simulink model "SerialCommIn_V2"  (R2017b)
settings: Solver=FixedStepAuto  StartTime=0.0  StopTime=inf  FixedStep=0.001  RelTol=1e-3  EnableMultiTasking=on
undefined symbols (not defined in the file): D10, D11, D12, D2, D5, D8, D9, PTA0, PTA2, PTB9, PTC4, PTD0, PTD2, PTD3
libraries: frdmk64flib x22, etargetslib x1
settings Model: ExtModeTrigDuration=5  Creator=montema2  LastModifiedBy=farona
settings OptimizationCC: PassReuseOutputArgsAs=Individual arguments  MaxStackSize=64
settings DebuggingCC: ParameterTunabilityLossMsg=error
settings HardwareCC: ProdBitPerPointer=32  ProdBitPerSizeT=32  ProdBitPerPtrDiffT=32  ProdLargestAtomicInteger=Long  ProdLargestAtomicFloat=Double  ProdWordSize=32  ProdHWDeviceType=ARM Compatible->ARM Cortex
settings SFSimCC: MATLABDynamicMemAlloc=off
settings RTWCC: SystemTargetFile=ert.tlc  HardwareBoard=NXP FRDM-K64F  TemplateMakefile=ert_default_tmf  GenerateReport=on  Toolchain=GNU Tools for ARM Embedded Processors  IncludeHyperlinkInReport=on  LaunchReport=on  GenerateTraceInfo=on  GenerateTraceReport=on  GenerateTraceReportSl=on  GenerateTraceReportSf=on  GenerateTraceReportEml=on
settings CodeAppCC: ForceParamTrailComments=on  IgnoreCustomStorageClasses=off  OperatorAnnotations=on  SimulinkDataObjDesc=on  SFDataObjDesc=on  InsertBlockDesc=on

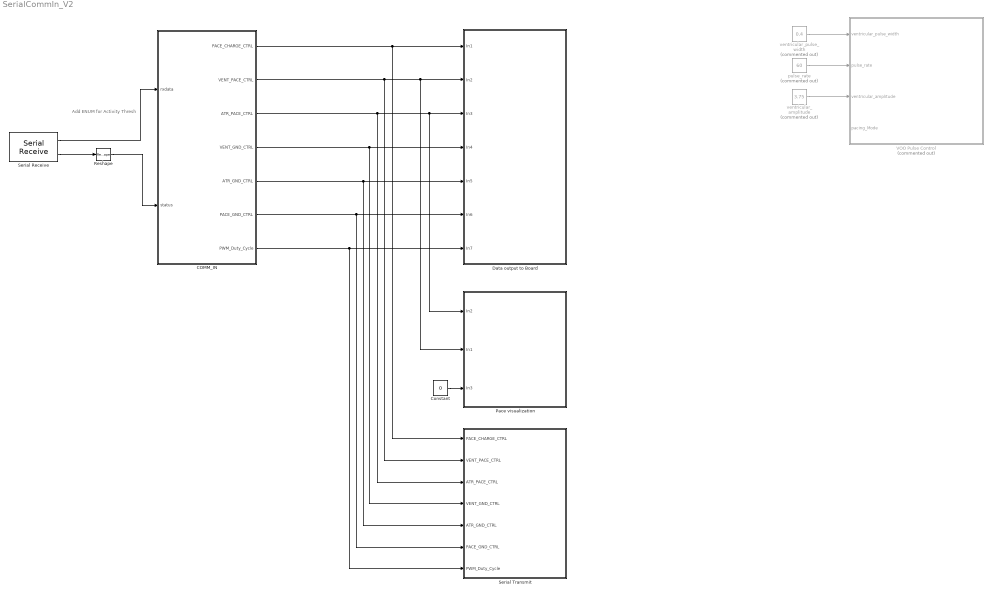
== system SerialCommIn_V2 ==
  note: Add ENUM for Activity Thresh
  COMM_IN : Stateflow chart  TreatAsAtomicUnit=on
  Constant : Constant  Value=0
  Data output to Board : Subsystem
  Pace visualization : Subsystem
  Reshape : Reshape  OutputDimensionality=Customize  OutputDimensions=[1]
  Serial Receive : frdmk64flib/Serial Receive  SCIModule=0  Baudrate=uint32(9600)  Parity=None  StopBits=1  HardwareFlowControl=None  ByteOrder=LittleEndian  DataType=uint8  DataLength=31  BlockingMode=off  OutputStatus=on  SampleTime=-1
      settings: SourceProductName=Simulink Coder Support Package for NXP FRDM-K64F Board
  Serial Transmit : Subsystem
  VOO Pulse Control : Subsystem  Commented=on
  pulse_rate : Constant  Commented=on  Value=60  OutMin=[50]  OutMax=[175]
  ventricular_amplitude : Constant  Commented=on  Value=3.75
  ventricular_pulse_width : Constant  Commented=on  Value=0.4
  wires:
  ventricular_pulse_width/1 -> VOO Pulse Control/1(ventricular_pulse_width)
  pulse_rate/1 -> VOO Pulse Control/2(pulse_rate)
  ventricular_amplitude/1 -> VOO Pulse Control/3(ventricular_amplitude)
  Serial Receive/2 -> Reshape/1
  COMM_IN/4(VENT_GND_CTRL) -> Serial Transmit/4(VENT_GND_CTRL), Data output to Board/4(In4)
  COMM_IN/6(PACE_GND_CTRL) -> Serial Transmit/6(PACE_GND_CTRL), Data output to Board/6(In6)
  COMM_IN/1(PACE_CHARGE_CTRL) -> Serial Transmit/1(PACE_CHARGE_CTRL), Data output to Board/1(In1)
  COMM_IN/7(PWM_Duty_Cycle) -> Serial Transmit/7(PWM_Duty_Cycle), Data output to Board/7(In7)
  COMM_IN/5(ATR_GND_CTRL) -> Serial Transmit/5(ATR_GND_CTRL), Data output to Board/5(In5)
  COMM_IN/2(VENT_PACE_CTRL) -> Serial Transmit/2(VENT_PACE_CTRL), Pace visualization/2(In1), Data output to Board/2(In2)
  COMM_IN/3(ATR_PACE_CTRL) -> Serial Transmit/3(ATR_PACE_CTRL), Pace visualization/1(In2), Data output to Board/3(In3)
  Serial Receive/1 -> COMM_IN/1(rxdata)
  Constant/1 -> Pace visualization/3(In3)
  Reshape/1 -> COMM_IN/2(status)

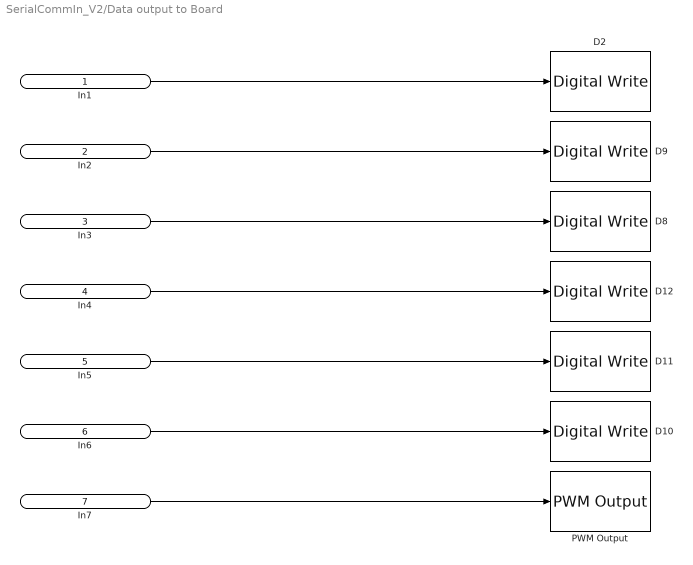
== system SerialCommIn_V2/Data output to Board ==
  In1 : Inport
  In2 : Inport  Port=2
  In3 : Inport  Port=3
  In4 : Inport  Port=4
  In5 : Inport  Port=5
  In6 : Inport  Port=6
  In7 : Inport  Port=7
  D10 : frdmk64flib/Digital Write  Whichpin=PTD0 (D10)
      settings: SourceProductName=Simulink Coder Support Package for NXP FRDM-K64F Board
  D11 : frdmk64flib/Digital Write  Whichpin=PTD2 (D11)
      settings: SourceProductName=Simulink Coder Support Package for NXP FRDM-K64F Board
  D12 : frdmk64flib/Digital Write  Whichpin=PTD3 (D12)
      settings: SourceProductName=Simulink Coder Support Package for NXP FRDM-K64F Board
  D2 : frdmk64flib/Digital Write  Whichpin=PTB9 (D2)
      settings: SourceProductName=Simulink Coder Support Package for NXP FRDM-K64F Board
  D8 : frdmk64flib/Digital Write  Whichpin=PTA0 (D8)
      settings: SourceProductName=Simulink Coder Support Package for NXP FRDM-K64F Board
  D9 : frdmk64flib/Digital Write  Whichpin=PTC4 (D9)
      settings: SourceProductName=Simulink Coder Support Package for NXP FRDM-K64F Board
  PWM Output : frdmk64flib/PWM Output  Whichpin=PTA2 (D5)  InitialFrequency=1000  InitialDutyCycle=0
      settings: SourceProductName=Simulink Coder Support Package for NXP FRDM-K64F Board
  wires:
  In1/1 -> D2/1
  In6/1 -> D10/1
  In2/1 -> D9/1
  In4/1 -> D12/1
  In3/1 -> D8/1
  In7/1 -> PWM Output/1
  In5/1 -> D11/1

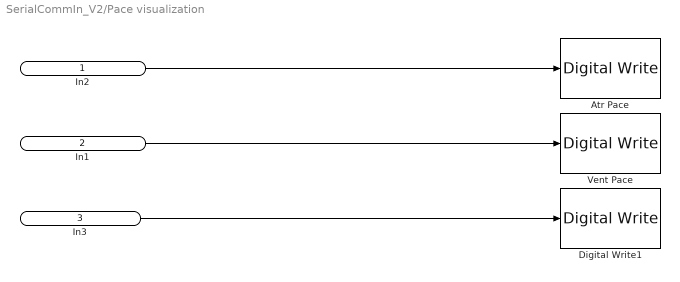
== system SerialCommIn_V2/Pace visualization ==
  In2 : Inport
  In1 : Inport  Port=2
  In3 : Inport  Port=3
  Atr Pace : frdmk64flib/Digital Write  Whichpin=GREEN_LED
      settings: SourceProductName=Simulink Coder Support Package for NXP FRDM-K64F Board
  Digital Write1 : frdmk64flib/Digital Write  Whichpin=BLUE_LED
      settings: SourceProductName=Simulink Coder Support Package for NXP FRDM-K64F Board
  Vent Pace : frdmk64flib/Digital Write  Whichpin=RED_LED
      settings: SourceProductName=Simulink Coder Support Package for NXP FRDM-K64F Board
  wires:
  In3/1 -> Digital Write1/1
  In2/1 -> Atr Pace/1
  In1/1 -> Vent Pace/1

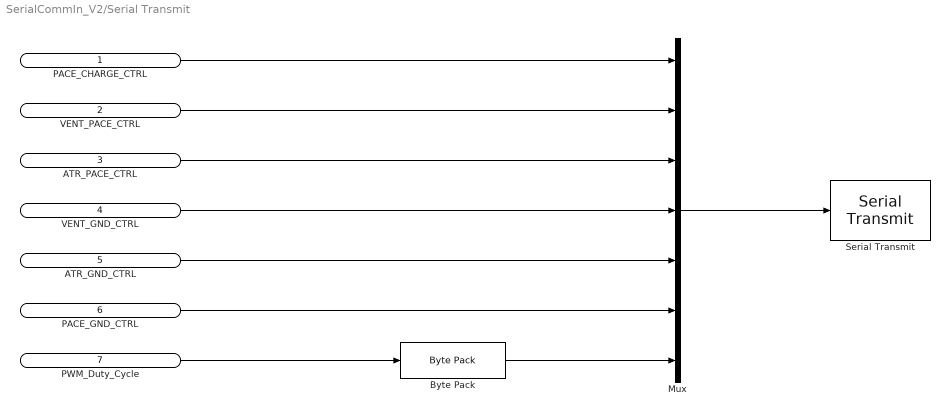
== system SerialCommIn_V2/Serial Transmit ==
  PACE_CHARGE_CTRL : Inport  OutDataTypeStr=boolean
  VENT_PACE_CTRL : Inport  Port=2  OutDataTypeStr=boolean
  ATR_PACE_CTRL : Inport  Port=3  OutDataTypeStr=boolean
  VENT_GND_CTRL : Inport  Port=4  OutDataTypeStr=boolean
  ATR_GND_CTRL : Inport  Port=5  OutDataTypeStr=boolean
  PACE_GND_CTRL : Inport  Port=6  OutDataTypeStr=boolean
  PWM_Duty_Cycle : Inport  Port=7  OutDataTypeStr=double
  Byte Pack : etargetslib/Byte Pack  datatypes={'double'}  byteAlign=1
  Mux : Mux  Inputs=7
  Serial Transmit : frdmk64flib/Serial Transmit  SCIModule=0  Baudrate=uint32(9600)  Parity=None  StopBits=1  HardwareFlowControl=None  ByteOrder=LittleEndian  BlockingMode=on  OutputStatus=off
      settings: SourceProductName=Simulink Coder Support Package for NXP FRDM-K64F Board
  wires:
  Mux/1 -> Serial Transmit/1
  PACE_CHARGE_CTRL/1 -> Mux/1
  VENT_PACE_CTRL/1 -> Mux/2
  ATR_PACE_CTRL/1 -> Mux/3
  VENT_GND_CTRL/1 -> Mux/4
  ATR_GND_CTRL/1 -> Mux/5
  PACE_GND_CTRL/1 -> Mux/6
  PWM_Duty_Cycle/1 -> Byte Pack/1
  Byte Pack/1 -> Mux/7

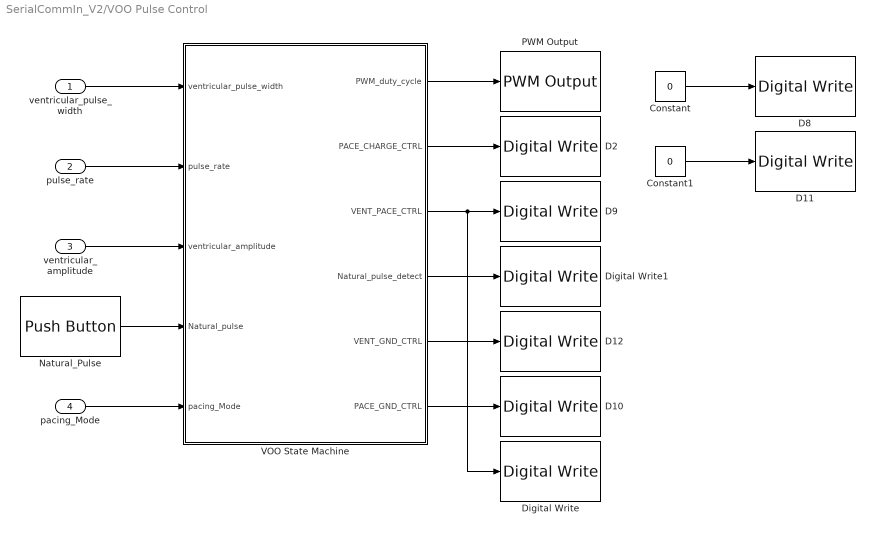
== system SerialCommIn_V2/VOO Pulse Control ==
  ventricular_pulse_width : Inport
  pulse_rate : Inport  Port=2
  ventricular_amplitude : Inport  Port=3
  pacing_Mode : Inport  Port=4
  Constant : Constant  Value=0
  Constant1 : Constant  Value=0
  D10 : frdmk64flib/Digital Write  Whichpin=PTD0 (D10)
      settings: SourceProductName=Simulink Coder Support Package for NXP FRDM-K64F Board
  D11 : frdmk64flib/Digital Write  Whichpin=PTD2 (D11)
      settings: SourceProductName=Simulink Coder Support Package for NXP FRDM-K64F Board
  D12 : frdmk64flib/Digital Write  Whichpin=PTD3 (D12)
      settings: SourceProductName=Simulink Coder Support Package for NXP FRDM-K64F Board
  D2 : frdmk64flib/Digital Write  Whichpin=PTB9 (D2)
      settings: SourceProductName=Simulink Coder Support Package for NXP FRDM-K64F Board
  D8 : frdmk64flib/Digital Write  Whichpin=PTA0 (D8)
      settings: SourceProductName=Simulink Coder Support Package for NXP FRDM-K64F Board
  D9 : frdmk64flib/Digital Write  Whichpin=PTC4 (D9)
      settings: SourceProductName=Simulink Coder Support Package for NXP FRDM-K64F Board
  Digital Write : frdmk64flib/Digital Write  Whichpin=RED_LED
      settings: SourceProductName=Simulink Coder Support Package for NXP FRDM-K64F Board
  Digital Write1 : frdmk64flib/Digital Write  Whichpin=BLUE_LED
      settings: SourceProductName=Simulink Coder Support Package for NXP FRDM-K64F Board
  Natural_Pulse : frdmk64flib/Push Button  Whichswitch=SW2  SampleTime1=-1
      settings: SourceProductName=Simulink Coder Support Package for NXP FRDM-K64F Board
  PWM Output : frdmk64flib/PWM Output  Whichpin=PTA2 (D5)  InitialFrequency=1000  InitialDutyCycle=0
      settings: SourceProductName=Simulink Coder Support Package for NXP FRDM-K64F Board
  VOO State Machine : Stateflow chart  TreatAsAtomicUnit=on
  wires:
  ventricular_pulse_width/1 -> VOO State Machine/1(ventricular_pulse_width)
  VOO State Machine/1(PWM_duty_cycle) -> PWM Output/1
  VOO State Machine/3(VENT_PACE_CTRL) -> Digital Write/1, D9/1
  pulse_rate/1 -> VOO State Machine/2(pulse_rate)
  VOO State Machine/2(PACE_CHARGE_CTRL) -> D2/1
  VOO State Machine/5(VENT_GND_CTRL) -> D12/1
  VOO State Machine/6(PACE_GND_CTRL) -> D10/1
  Constant/1 -> D8/1
  Constant1/1 -> D11/1
  Natural_Pulse/1 -> VOO State Machine/4(Natural_pulse)
  VOO State Machine/4(Natural_pulse_detect) -> Digital Write1/1
  ventricular_amplitude/1 -> VOO State Machine/3(ventricular_amplitude)
  pacing_Mode/1 -> VOO State Machine/5(pacing_Mode)

== stateflow chart SerialCommIn_V2/COMM_IN ==
  state INITIAL
    %Set intial values of parameters
    %VOO mode?
    entry: rateAdapt = 0;
    vent_Pulse_Width = 10; %milliseconds
    atr_Pulse_Width = 10;
    min_Rate_Lim = 60; %bpm
    vent_Pulse_Amp = 3.5; %volts
    atr_Pulse_Amp = 3.5;
  state VENT_CURRENT_IN
    entry:PWM_Duty_Cycle = vent_Pulse_Amp;
    PACE_CHARGE_CTRL=false;
    VENT_GND_CTRL=false;
    VENT_PACE_CTRL=true;
  state STANDBY
    %Wait for signal from DCM
  state VENTRICLE_INIT
    entry:VENT_PACE_CTRL=false;
    VENT_GND_CTRL=true;
    ATR_PACE_CTRL=false;
    ATR_GND_CTRL=true;
    PACE_CHARGE_CTRL=true;
    PACE_GND_CTRL=true;
  note: double check ATR_GND_CTRL state
  state VENT_PULSE_SENSE [commented out]
  note: double check VENT_GND_CTRL state
  state ATRIAL_INIT
    entry:VENT_PACE_CTRL=false;
    VENT_GND_CTRL=true;
    ATR_PACE_CTRL=false;
    ATR_GND_CTRL=true;
    PACE_CHARGE_CTRL=true;
    PACE_GND_CTRL=true;
  state PARAM_INIT
    entry: pace_Mode = rxdata(1);
    min_Rate_Lim = rxdata(2);
    max_Rate_Lim = rxdata(3);
    max_Sensor_Rate = rxdata(4);
    fix_AV_Delay = rxdata(5);
    dyn_AV_Delay = rxdata(6);
    min_Dyn_AV_Delay = rxdata(7);
    sensed_AV_Delay_Offset_State = rxdata(8);
    sensed_AV_Delay_Offset_Val = rxdata(9);
    vent_Pulse_Amp = ((rxdata(10)/5)*100);
    atr_Pulse_Amp = ((rxdata(11)/5)*100);
    vent_Pulse_Width = rxdata(12);
    atr_Pulse_Width = rxdata(13);
    vent_Sens = rxdata(14);
    atr_Sens = rxdata(15);
    vent_Ref_Per = rxdata(16);
    atr_Ref_Per = rxdata(17);
    PVARP = rxdata(18);
    PVARP_Ext_State = rxdata(19);
    PVARP_Ext_Val = rxdata(20);
    hyst_State = rxdata(21);
    hyst_Rate_Lim = rxdata(22);
    rate_Smooth_State = rxdata(23);
    rate_Smooth_Val = rxdata(24);
    ATR_State = rxdata(25);
    ATR_Duration = rxdata(26);
    ATR_Fallback = rxdata(27);
    activity_Thresh = rxdata(28);
    reaction_Time = rxdata(29);
    response_Factor = rxdata(30);
    recovery_Time = rxdata(31);
  state VENT_CURRENT_OUT
    entry:
    VENT_PACE_CTRL=false;
    PACE_CHARGE_CTRL=true;
    VENT_GND_CTRL=true;
  state VVI_INIT [commented out]
    entry:VENT_PACE_CTRL=false;
    VENT_GND_CTRL=true;
    PACE_CHARGE_CTRL=true;
    PACE_GND_CTRL=true;
  state AAI_INIT [commented out]
    entry:ATR_PACE_CTRL=false;
    ATR_GND_CTRL=true;
    PACE_CHARGE_CTRL=true;
    PACE_GND_CTRL=true;
  state ATR_CURRENT_IN
    entry:PWM_Duty_Cycle = atr_Pulse_Amp;
    PACE_CHARGE_CTRL=false;
    ATR_GND_CTRL=false;
    ATR_PACE_CTRL=true;
  state DUAL_INIT
    entry:VENT_PACE_CTRL=false;
    VENT_GND_CTRL=true;
    ATR_PACE_CTRL=false;
    ATR_GND_CTRL=true;
    PACE_CHARGE_CTRL=true;
    PACE_GND_CTRL=true;
  state ATR_PULSE_SENSE [commented out]
  state DDD_INIT
  state ATR_CURRENT_OUT
    entry:
    ATR_PACE_CTRL=false;
    PACE_CHARGE_CTRL=true;
    ATR_GND_CTRL=true;
  (default) -> INITIAL
  INITIAL -> STANDBY
  ATR_CURRENT_OUT -> VENT_CURRENT_IN [order 2] : [(pace_Mode ==  5 || pace_Mode ==11)&&(after((fix_AV_Delay),msec))]
  VENTRICLE_INIT -> VENT_CURRENT_IN : [after(((min_Rate_Lim)*1000),msec)]
  VENT_CURRENT_IN -> VENT_PULSE_SENSE [commented out] : [(natural_Pace == 1)&&(pace_Mode == 3|| pace_Mode == 4 || pace_Mode == 6 || pace_Mode == 9 || pace_Mode == 10 || pace_Mode == 12)]
  (junction 5) -> STANDBY [order 2]
  STANDBY -> (junction 5) : [status == 0]
  VENT_CURRENT_OUT -> VENT_CURRENT_IN [order 1] : [(pace_Mode == 1 || pace_Mode ==3 || pace_Mode == 7 || pace_Mode == 9)&&(after(((60/min_Rate_Lim)*1000)-(vent_Pulse_Width),msec))]
  VENT_CURRENT_IN -> VENT_CURRENT_OUT : [after((vent_Pulse_Width),msec)]
  (junction 7) -> VENTRICLE_INIT [order 1] : [pace_Mode ==1 || pace_Mode == 3 || pace_Mode ==7 || pace_Mode == 9]
  (junction 5) -> (junction 38) [order 1] : [rxdata(0) > 0 && rxdata(1) < 13 ]
  (junction 38) -> PARAM_INIT : [rxdata(0) > 6]{rateAdapt = 1}
  VENT_CURRENT_OUT -> VENT_PULSE_SENSE [commented out]
  ATRIAL_INIT -> ATR_CURRENT_IN : [after(((min_Rate_Lim)*1000),msec)]
  (junction 7) -> ATRIAL_INIT [order 2] : [pace_Mode ==2 || pace_Mode == 4 || pace_Mode ==8 || pace_Mode ==10]
  (junction 7) -> VVI_INIT [commented out] : [pace_Mode ==3 || pace_Mode == 9]
  PARAM_INIT -> (junction 7)
  (junction 7) -> AAI_INIT [commented out] : [pace_Mode ==4 || pace_Mode ==10 ]
  VENT_CURRENT_OUT -> ATR_CURRENT_IN [order 2] : [(pace_Mode ==  5 || pace_Mode ==11)&&(after(((60/min_Rate_Lim)*1000)-(vent_Pulse_Width)-(atr_Pulse_Width)-(fix_AV_Delay),msec))]
  (junction 7) -> DUAL_INIT [order 3] : [pace_Mode ==5 || pace_Mode == 11]
  (junction 7) -> DDD_INIT [order 4] : [pace_Mode ==6 || pace_Mode ==12 ]
  DUAL_INIT -> ATR_CURRENT_IN : [after(((min_Rate_Lim)*1000),msec)]
  DDD_INIT -> ATR_CURRENT_IN : [after(((min_Rate_Lim)*1000),msec)]
  ATR_CURRENT_OUT -> ATR_CURRENT_IN [order 1] : [(pace_Mode == 2 || pace_Mode == 4 || pace_Mode == 8 || pace_Mode == 10)&&(after(((60/min_Rate_Lim)*1000)-(atr_Pulse_Width),msec)) ]
  ATR_CURRENT_IN -> ATR_CURRENT_OUT : [after((atr_Pulse_Width),msec)]
  data: rxdata input uint8; status input uint8; PACE_CHARGE_CTRL output boolean; VENT_PACE_CTRL output boolean; ATR_PACE_CTRL output boolean; VENT_GND_CTRL output boolean; ATR_GND_CTRL output boolean; PACE_GND_CTRL output boolean; PWM_Duty_Cycle output single; natural_Pace local; sensed_AV_Delay_Offset_State local boolean; sensed_AV_Delay_Offset_Val local int16; atr_Sens local single; PVARP local uint16; ATR_Fallback local uint16; activity_Thresh local Enum: <class name>; recovery_Time local uint16; response_Factor local uint16; reaction_Time local uint16; max_Rate_Lim local uint16; max_Sensor_Rate local uint16; min_Dyn_AV_Delay local uint16; dyn_AV_Delay local boolean; vent_Ref_Per local uint16; vent_Sens local single; atr_Ref_Per local uint16; hyst_State local boolean; PVARP_Ext_State local boolean; PVARP_Ext_Val local uint16; rate_Smooth_Val local uint16; ATR_State local boolean; hyst_Rate_Lim local uint16; rate_Smooth_State local boolean; ATR_Duration local uint16; rateAdapt local; pace_Mode local Enum: pacing_Mode.m =0; fix_AV_Delay local uint16; atr_Pulse_Width local uint16; vent_Pulse_Width local; min_Rate_Lim local uint16; vent_Pulse_Amp local single; atr_Pulse_Amp local single

== stateflow chart SerialCommIn_V2/VOO Pulse Control/VOO State Machine ==
  note: Switch States:
      | true=closed
      | false=open
  state current_into_heart
    entry:
    PACE_CHARGE_CTRL=false;
    VENT_GND_CTRL=false;
    VENT_PACE_CTRL=true;
  state start_state
    entry:VENT_PACE_CTRL=false;
    VENT_GND_CTRL=true;
    PACE_CHARGE_CTRL=true;
    PACE_GND_CTRL=true;
    PWM_duty_cycle=((ventricular_amplitude/5)*100);
  state current_out_of_heart
    entry:
    VENT_PACE_CTRL=false;
    PACE_CHARGE_CTRL=true;
    VENT_GND_CTRL=true;
  state natural_pace
    entry: Natural_pulse_detect=true;
    exit: Natural_pulse_detect=false;
  (default) -> start_state
  start_state -> current_into_heart [order 1] : [after(((60/pulse_rate)*1000),msec)]
  current_into_heart -> natural_pace [order 2] : [Natural_pulse==true]
  start_state -> natural_pace [order 2] : [Natural_pulse==true]
  natural_pace -> start_state : [Natural_pulse==false]
  current_into_heart -> current_out_of_heart [order 1] : [after((ventricular_pulse_width),msec)]
  current_out_of_heart -> current_into_heart [order 1] : [after(((60/pulse_rate)*1000)-(ventricular_pulse_width),msec)]
  current_out_of_heart -> natural_pace [order 2] : [Natural_pulse==true]
  data: ventricular_pulse_width input double; pulse_rate input double; ventricular_amplitude input double; PWM_duty_cycle output double [0..100]; PACE_CHARGE_CTRL output boolean; VENT_PACE_CTRL output boolean; Natural_pulse_detect output; VENT_GND_CTRL output boolean; PACE_GND_CTRL output boolean; Natural_pulse input boolean; pacing_Mode input uint8
